simulink model "AF_Simulink1"  (R2022b)
settings: Solver=VariableStepAuto  StartTime=0.0  StopTime=10.0  RelTol=1e-3
libraries: aerolib6dof2 x1
settings Model: Creator=matho  LastModifiedBy=matho

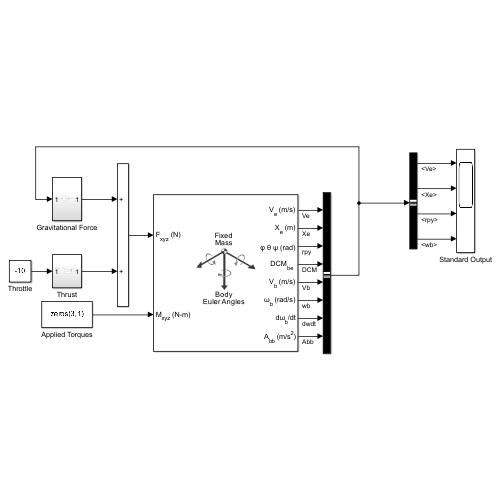
[thumbnail: Simulink's stored preview of the top-level diagram]
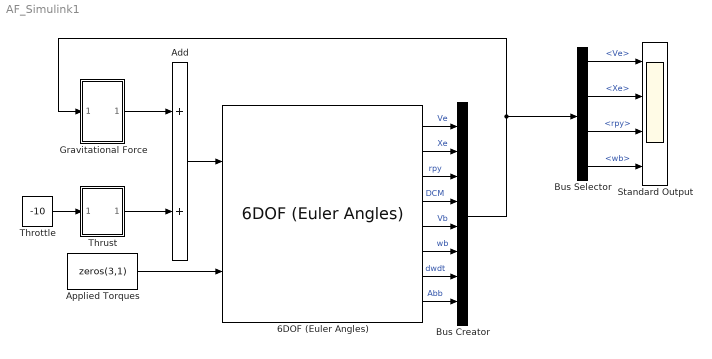
== system AF_Simulink1 ==
  6DOF (Euler Angles) : aerolib6dof2/6DOF (Euler Angles)  units=Metric (MKS)  mtype=Fixed  rep=Euler Angles  xme_0=[0 0 0]  Vm_0=[0 0 0]  eul_0=[0 0 0]  pm_0=[0 0 0]  mass_0=1.0  mass_e=0.5  mass_f=2.0  inertia=eye(3)  inertia_e=eye(3)  inertia_f=2*eye(3)  k_quat=1.0  vre_flag=on  abi_flag=off  aMode=0  xme_statename=''  Vm_statename=''  eul_statename=''  quat_statename=''  pm_statename=''  mass_statename=''
  Add : Sum
  Applied Torques : Constant  Value=zeros(3,1)
  Bus Creator : BusCreator  Inputs=8
  Bus Selector : BusSelector  OutputSignals=Ve,Xe,rpy,wb
  Gravitational Force : Subsystem
  Standard Output : Scope  NumInputPorts=4
  Throttle : Constant  Value=-10
  Thrust : Subsystem
  wires:
  6DOF (Euler Angles)/1 -> Bus Creator/1  "Ve"
  6DOF (Euler Angles)/2 -> Bus Creator/2  "Xe"
  6DOF (Euler Angles)/3 -> Bus Creator/3  "rpy"
  6DOF (Euler Angles)/4 -> Bus Creator/4  "DCM"
  6DOF (Euler Angles)/5 -> Bus Creator/5  "Vb"
  6DOF (Euler Angles)/6 -> Bus Creator/6  "wb"
  6DOF (Euler Angles)/7 -> Bus Creator/7  "dwdt"
  6DOF (Euler Angles)/8 -> Bus Creator/8  "Abb"
  Bus Creator/1 -> Gravitational Force/1(In1), Bus Selector/1
  Gravitational Force/1(Out1) -> Add/1
  Applied Torques/1 -> 6DOF (Euler Angles)/2
  Bus Selector/1 -> Standard Output/1  "<Ve>"
  Bus Selector/2 -> Standard Output/2  "<Xe>"
  Bus Selector/3 -> Standard Output/3  "<rpy>"
  Bus Selector/4 -> Standard Output/4  "<wb>"
  Add/1 -> 6DOF (Euler Angles)/1
  Throttle/1 -> Thrust/1(In1)
  Thrust/1(Out1) -> Add/2

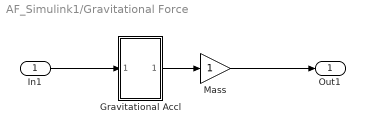
== system AF_Simulink1/Gravitational Force ==
  In1 : Inport
  Gravitational Accl : Subsystem
  Mass : Gain
  Out1 : Outport
  wires:
  Mass/1 -> Out1/1
  Gravitational Accl/1(Out1) -> Mass/1
  In1/1 -> Gravitational Accl/1(In1)

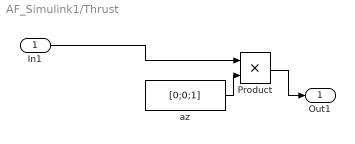
== system AF_Simulink1/Thrust ==
  In1 : Inport
  Product : Product
  az : Constant  Value=[0;0;1]
  Out1 : Outport
  wires:
  az/1 -> Product/2
  Product/1 -> Out1/1
  In1/1 -> Product/1

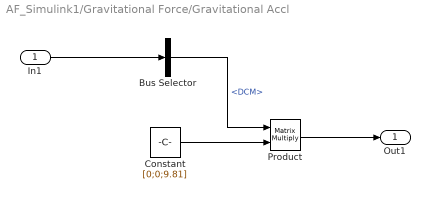
== system AF_Simulink1/Gravitational Force/Gravitational Accl ==
  In1 : Inport
  Bus Selector : BusSelector  OutputSignals=DCM
  Constant : Constant  Value=[0;0;9.81]
  Product : Product  Multiplication=Matrix(*)
  Out1 : Outport
  wires:
  Constant/1 -> Product/2
  In1/1 -> Bus Selector/1
  Product/1 -> Out1/1
  Bus Selector/1 -> Product/1  "<DCM>"
